simulink model "localization_and_state_estimation"  (R2023a)
settings: Solver=ode1  StartTime=0.0  StopTime=inf  FixedStep=1/60  RelTol=1e-3  EnableMultiTasking=on
model workspace (MAT data in the model file):
  downCamStepSize = Simulink.Parameter
  downCamStepSize.Value = Simulink.data.Expression
  downCamStepSize.Value.ExpressionString = "qc_get_step_size*ceil(1/60/qc_get_step_size)"
  downCamStepSize.DataType = 'auto'
  downCamStepSize.Complexity = 'real'
  downCamStepSize.Dimensions = -1
  lidarStepSize = Simulink.Parameter
  lidarStepSize.Value = Simulink.data.Expression
  lidarStepSize.Value.ExpressionString = "qc_get_step_size*ceil(1/5/qc_get_step_size)"
  lidarStepSize.DataType = 'auto'
  lidarStepSize.Complexity = 'real'
  lidarStepSize.Dimensions = -1
  mainStepSize = Simulink.Parameter
  mainStepSize.Value = Simulink.data.Expression
  mainStepSize.Value.ExpressionString = "qc_get_step_size"
  mainStepSize.DataType = 'auto'
  mainStepSize.Complexity = 'real'
  mainStepSize.Dimensions = -1
  mode = Simulink.Parameter
  mode.Value = 1
  mode.Description = '0 - education speeds via wheel speed commands
    | 1 - education speeds via body speed commands
    | 2 - research speeds via wheel speed commands
    | 3 - research speeds via body speed commands'
  mode.DataType = 'auto'
  mode.Complexity = 'real'
  mode.Dimensions = [1 1]
  realSenseStepSize = Simulink.Parameter
  realSenseStepSize.Value = Simulink.data.Expression
  realSenseStepSize.Value.ExpressionString = "qc_get_step_size*ceil(1/30/qc_get_step_size)"
  realSenseStepSize.DataType = 'auto'
  realSenseStepSize.Complexity = 'real'
  realSenseStepSize.Dimensions = -1
undefined symbols (not defined in the file): gcbh, JPEG, Point, video_display_show
libraries: quarc_library x33, simulink x2
(part 1 of 2)
settings Model: SimulationMode=external  ExtModeTrigDuration=10000  Creator=mbohra  LastModifiedBy=mbohra
settings SolverCC: AlgebraicLoopSolver=TrustRegion  PositivePriorityOrder=on
settings DataIOCC: ReturnWorkspaceOutputs=off
settings DebuggingCC: ParameterPrecisionLossMsg=none  UnconnectedInputMsg=warning  UnconnectedOutputMsg=warning  UnconnectedLineMsg=warning  ArithmeticOperatorsInVariantConditions=warning
settings HardwareCC: ProdBitPerLong=64  ProdLargestAtomicInteger=LongLong  ProdLargestAtomicFloat=Double  ProdLongLongMode=on  ProdHWDeviceType=ARM Compatible->ARM 64-bit (LP64)
settings ModelReferenceCC: EnableRefExpFcnMdlSchedulingChecks=on
settings SFSimCC: SimUseLocalCustomCode=off  CustomCodeUndefinedFunction=UseInterfaceOnly
settings RTWCC: Description=QUARC Linux QBot Platform Target Using Toolchain  SystemTargetFile=quarc_linux_qbot_platform.tlc  TemplateMakefile=quarc_default_tmf  RTWUseLocalCustomCode=off  Toolchain=QUARC linux_qbot_platform | gmake (64-bit Windows)  BuildConfiguration=Faster Runs
settings CodeAppCC: StateflowObjectComments=on
settings STFCustomTargetCC: SystemTargetFile=quarc_linux_qbot_platform.tlc
settings GRTTargetCC: ParMdlRefBuildCompliant=off  CompOptLevelCompliant=off  CombineOutputUpdateFcns=off  MatFileLogging=off  CPPClassGenCompliant=off  GRTInterface=on  ExtMode=on  ExtModeMexFile=quarc_comm  ExtModeMexArgs='-w -d /tmp -uri %u','tcpip://192.168.3.14:17001'
settings ConfigComp: CovMetricSettings=dswe

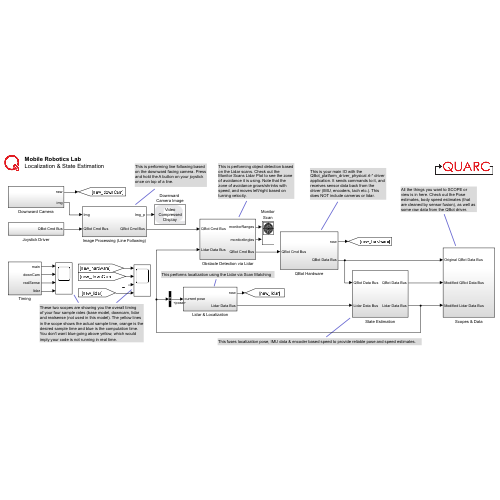
[thumbnail: Simulink's stored preview of the top-level diagram]
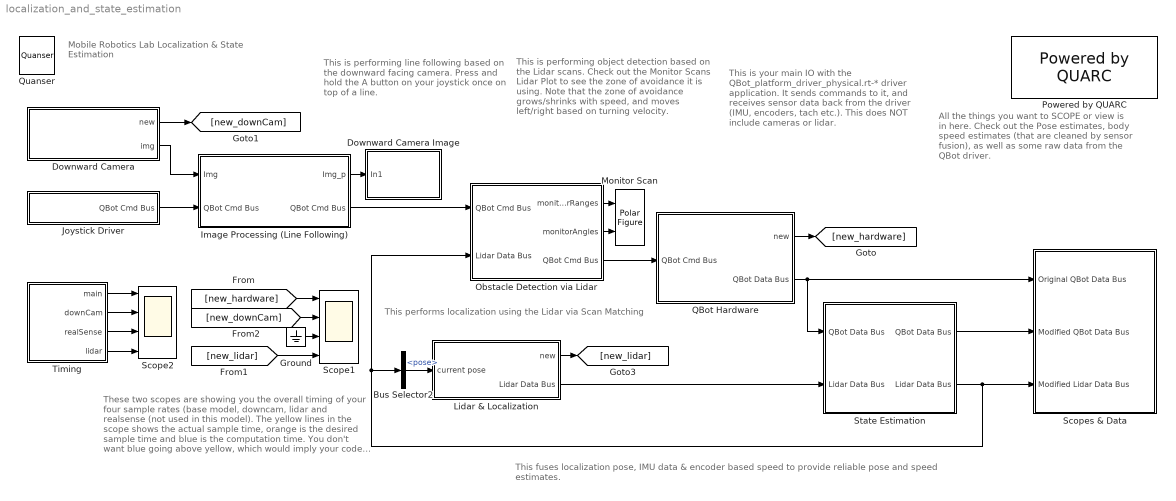
== system localization_and_state_estimation ==
  note: These two scopes are showing you the overall timing
      | of your four sample rates (base model, downcam, lidar
      | and realsense (not used in this model). The yellow lines
      | in the scope shows the actual sample time, orange is the
      | desired sample time and blue is the computation time.
      | You don't want blue going above yellow, which would
      | imply your code is not running in real time.
  note: This is performing line following based on the downward facing camera. Press and hold the A button on your joystick once on top of a line.
  note: Mobile Robotics Lab
      | Localization & State Estimation
  note: This is performing object detection based on the Lidar scans. Check out the Monitor Scans Lidar Plot to see the zone of avoidance it is using. Note that the zone of avoidance grows/shrinks with speed, and moves left/right based on turning velocity.
  note: This is your main IO with the QBot_platform_driver_physical.rt-* driver application. It sends commands to it, and receives sensor data back from the driver (IMU, encoders, tach etc.). This does NOT include cameras or lidar.
  note: All the things you want to SCOPE or view is in here. Check out the Pose estimates, body speed estimates (that are cleaned by sensor fusion), as well as some raw data from the QBot driver.
  note: This performs localization using the Lidar via Scan Matching
  note: This fuses localization pose, IMU data & encoder based speed to provide reliable pose and speed estimates.
  Bus Selector2 : BusSelector  OutputSignals=pose
  Downward Camera Image : Subsystem  LoadFcn=set_param(gcbh, 'UserData', gcb);  StartFcn=video_display_show([gcb, '/Video Display'], 'add', gcb);  mask(Video Compressed Display){algorithm=JPEG, quality=50, sample_time=-1, use_hardware=on}
      mask prompts: algorithm "Compression algorithm:"; quality "Compression quality (0-100):"; sample_time "Sample time (seconds):"; use_hardware "Use hardware acceleration for video display"
      mask help: Displays a video stream on the host, using compression to minimize bandwidth.
      mask init:
      | qc_set_display('Video\nCompressed\nDisplay');
      settings: UndoDeleteFcn=set_param(gcbh, 'UserData', gcb);  OpenFcn=video_display_show([gcb, '/Video Display'], 'show', gcb);  PreDeleteFcn=video_display_show([gcb, '/Video Display'], 'delete');
      settings: CopyFcn=|
      | set_param(gcbh, 'UserData', gcb);
      | set_param(gcbh, 'LinkStatus', 'none');
      settings: NameChangeFcn=|
      | video_display_show([get_param(gcbh, 'UserData'), '/Video Display'], 'rename', [gcb, '/Video Display']);
      | video_display_show([gcb, '/Video Display'], 'add', gcb);
      | set_param(gcbh, 'UserData', gcb);
      mask Help: web(qc_get_block_help_path(gcb));
      mask TypeOptions algorithm: Image Compress/algorithm
      mask TypeOptions quality: Image Compress/quality
      mask TypeOptions sample_time: Video Display/sample_time
      mask TypeOptions use_hardware: Video Display/use_hardware
      mask Display:
      | patch([0.98591 0.98591 0.62618 0.59072 0.56147   0.536   0.536  0.5441 0.56912 0.59207 0.60881 0.62276 0.63527 0.64364  0.6485  0.6485 0.64706 0.64499 0.63662 0.62411 0.61232 0.59837 0.58307 0.56147   0.536   0.536  0.5441  0.5747 0.60953 0.63662 0.67001  0.7034 0.72851 0.75425 0.77927 0.80294 0.82454 0.84119 0.85865 0.87395 0.88574 0.89339  0.8969 0.89969 0.89969 0.89267  0.8816 0.87044 0.85649  0.8384 0.81824 0.80294 0.78764 0.77513 0.76676 0.75776 0.76397 0.77513 0.79178 0.80987 0.82796 0.84326 0.86207 0.98528],[0.18689 0.05522 0.05522 0.05171 0.05171    0.05 0.18338 0.18338 0.19148 0.20435 0.22298 0.24863 0.28589 0.33125 0.38138 0.55139 0.59801 0.63761 0.68189 0.72149 0.74939 0.76694 0.77855 0.79367 0.79952 0.92768 0.92768 0.92768 0.92417 0.92066 0.91364  0.9032 0.89384 0.88106 0.86594 0.85073 0.82634 0.80537 0.77855 0.74363 0.70403 0.65858 0.61079 0.59099 0.41513 0.37202 0.31847 0.29048 0.25556 0.23342  0.2102 0.19382 0.18221 0.17285 0.16943 0.16124  0.1589 0.16241 0.16709 0.17168  0.1787 0.18221 0.18689 0.18689],[0.9,0.90,0.91])
      | patch([0.536 0.52601 0.46823 0.44528 0.41603 0.39101 0.35555 0.33116 0.31451 0.29291  0.2804 0.26717 0.25322 0.23999 0.22406 0.20732 0.19337 0.17528 0.15935 0.14396 0.13217 0.11759 0.10922 0.10085 0.09671 0.09392 0.09041 0.08906 0.08906 0.09464  0.0995 0.10778 0.11894 0.13145 0.14675 0.16349 0.17672 0.19409 0.20732 0.22406 0.23999 0.26159 0.27833 0.29849 0.31793 0.33602 0.35411 0.37085 0.39245 0.41603   0.536   0.536 0.53159 0.46409   0.446 0.42026 0.39587 0.37571 0.36113 0.34925 0.34088 0.33809 0.33809 0.34088 0.34583 0.35627 0.36392 0.38129 0.39587 0.41117 0.42719 0.44672  0.4676 0.48353 0.48353 0.52394   0.536],[0.05 0.04829 0.04712 0.04712 0.04829 0.05063 0.05405 0.05873 0.06107 0.06692 0.07043 0.07619 0.08087 0.08672 0.09482 0.10652 0.11696 0.13325  0.1508 0.17168 0.19499 0.22415 0.25439 0.28472 0.31379 0.35456 0.38489 0.41513 0.58055 0.63878 0.68774 0.72149 0.75641 0.78089 0.80537 0.82859 0.84029 0.85658 0.86594 0.87404  0.8834 0.89267 0.90086 0.90788 0.91247 0.91832 0.92066   0.923 0.92651 0.92768 0.92768 0.79952 0.79952 0.79952 0.79718 0.78899 0.77153 0.75056 0.72149 0.68072 0.62249  0.5549 0.41396 0.37085 0.33242 0.28121 0.25205 0.22181 0.20552 0.19499 0.18572 0.18221 0.17753 0.17636 0.17753  0.1787  0.1787],[0.9,0.90,0.91])
      | disp('Video\nCompressed\nDisplay');
  Downward Camera : Subsystem
  Ground : Ground
  Image Processing (Line Following) : Subsystem
  Joystick Driver : Subsystem
  Lidar & Localization : Subsystem
  Monitor Scan : quarc_library/Sinks/Figures/Polar Figure  figure_mode=Use figure window  figure_tag=figure1  axes_tag=axes1  plot_mode=Frame-based  minimum_rho=0  maximum_rho=4  minimum_theta=0  maximum_theta=360  zero_location=top  direction=counterclockwise  buffer_size=2  update_rate=1  sample_time=-1  initial_position="1290    55   483   448"  initial_visibility=off  line1_style=None  line1_width=0.5  line1_color=[0 0 0]  marker1=Point (.)  marker1_size=6  marker1_edge_color=[0 0 0]  marker1_face_color=[0 0 0]  line2_style=Solid line (-)  line2_width=0.5  line2_color=[0.85098 0.32549 0.0980392]  marker2=None  marker2_size=6  marker2_edge_color=[0.85098 0.32549 0.0980392]  marker2_face_color=[0.85098 0.32549 0.0980392]  line3_style=Solid line (-)  line3_width=0.5  line3_color=[0.929412 0.694118 0.12549]  marker3=None  marker3_size=6  marker3_edge_color=[0.929412 0.694118 0.12549]  marker3_face_color=[0.929412 0.694118 0.12549]  line4_style=Solid line (-)  line4_width=0.5  line4_color=[0.494118 0.184314 0.556863]  marker4=None  marker4_size=6  marker4_edge_color=[0.494118 0.184314 0.556863]  marker4_face_color=[0.494118 0.184314 0.556863]  line5_style=Solid line (-)  line5_width=0.5  line5_color=[0.466667 0.67451 0.188235]  marker5=None  marker5_size=6  marker5_edge_color=[0.466667 0.67451 0.188235]  marker5_face_color=[0.466667 0.67451 0.188235]
      settings: SourceProductName=QUARC Targets
  Obstacle Detection via Lidar : Subsystem
  Powered by QUARC : quarc_library/Logos/Powered by QUARC
  QBot Hardware : Subsystem
  Quanser : quarc_library/Logos/Quanser
  Scope1 : Scope  NumInputPorts=4
  Scope2 : Scope  NumInputPorts=4
  Scopes & Data : Subsystem
  State Estimation : Subsystem
  Timing : Subsystem
  wires:
  QBot Hardware/2(QBot Data Bus) -> Scopes & Data/1(Original QBot Data Bus), State Estimation/1("QBot Data Bus ")
  QBot Hardware/1(new) -> [new_hardware]
  Lidar & Localization/1(new) -> [new_lidar]
  [new_downCam] -> Scope1/2
  Timing/3(realSense) -> Scope2/3
  Timing/4(lidar) -> Scope2/4
  [new_lidar] -> Scope1/4
  Timing/2(downCam) -> Scope2/2
  [new_hardware] -> Scope1/1
  Timing/1(main) -> Scope2/1
  Obstacle Detection via Lidar/1(monitorRanges) -> Monitor Scan/1
  Obstacle Detection via Lidar/2(monitorAngles) -> Monitor Scan/2
  Obstacle Detection via Lidar/3(QBot Cmd Bus) -> QBot Hardware/1(QBot Cmd Bus)
  Downward Camera/2(img) -> Image Processing (Line Following)/1(Img)
  Joystick Driver/1(QBot Cmd Bus) -> Image Processing (Line Following)/2(QBot Cmd Bus)
  Image Processing (Line Following)/1(Img_p) -> Downward Camera Image/1(In1)
  Image Processing (Line Following)/2(" QBot Cmd Bus") -> Obstacle Detection via Lidar/1("QBot Cmd Bus ")
  Downward Camera/1(new) -> [new_downCam]
  Ground/1 -> Scope1/3
  Lidar & Localization/2(Lidar Data Bus) -> State Estimation/2("Lidar Data Bus ")
  State Estimation/2(Lidar Data Bus) -> Bus Selector2/1, Obstacle Detection via Lidar/2(Lidar Data Bus), Scopes & Data/3(Modified Lidar Data Bus)
  Bus Selector2/1 -> Lidar & Localization/1(current pose)  "<pose>"
  State Estimation/1(QBot Data Bus) -> Scopes & Data/2(Modified QBot Data Bus)

== system localization_and_state_estimation/Downward Camera Image ==
  In1 : Inport
  Channel : quarc_library/Signal Routing/Channel  channel=0  buffer_size=1
  Image Compress : quarc_library/Image Processing/Generic/Image Compress  algorithm=JPEG  source=Internal dialog parameter  quality=quality  output_dim=-1
  Video Display : quarc_library/Multimedia/Video Display  Tag="localization_and_state_estimation/Downward  Camera Image/Video Display"  sample_time=sample_time  use_hardware=on
  wires:
  Channel/1 -> Video Display/1
  In1/1 -> Image Compress/1
  Image Compress/1 -> Channel/1

== system localization_and_state_estimation/Downward Camera ==
  Rate Transition : RateTransition
  Video Capture : quarc_library/Multimedia/Video Capture  source=device  device=0  filename=sample_movie.mov  value=[0 0; 0 0]  resolution=640 x 400  width=640  height=400  output_format=MATLAB greyscale (HxW)  data_type=uint8  sample_time=downCamStepSize  brightness_override=off  brightness=50.0  contrast_override=off  contrast=50.0  hue_override=off  hue=50.0  saturation_override=off  saturation=50.0  sharpness_override=off  sharpness=50.0  gamma_override=off  gamma=50.0  coloreffect_override=off  coloreffect=None  whitebalance_override=off  whitebalance=50.0  backlightcompensation_override=off  backlightcompensation=0.0  gain_override=on  gain=17.0  pan_override=off  pan=50.0  tilt_override=off  tilt=50.0  roll_override=off  roll=50.0  zoom_override=off  zoom=0.0  exposure_override=on  exposure=39.0  iris_override=off  iris=50.0  mirror_override=off  mirror=None  focus_override=off  focus=0.0
      settings: SourceProductName=QUARC Targets
  new : Outport
  img : Outport  Port=2
  wires:
  Video Capture/2 -> Rate Transition/1
  Video Capture/1 -> img/1
  Rate Transition/1 -> new/1

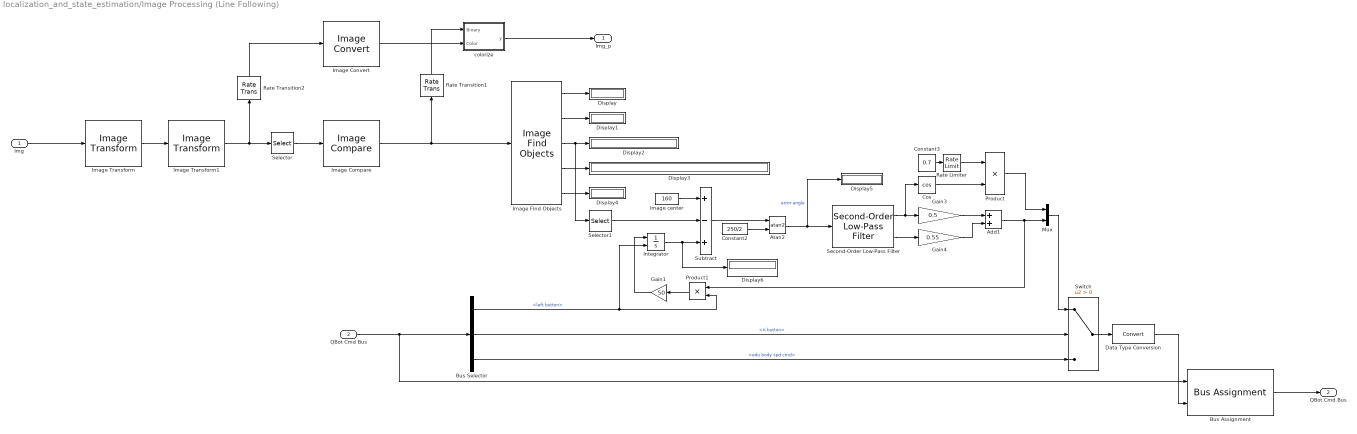
== system localization_and_state_estimation/Image Processing (Line Following) ==
  Img : Inport
  QBot Cmd Bus : Inport  Port=2
  Add1 : Sum
  Atan2 : Trigonometry  Operator=atan2
  Bus Assignment : BusAssignment  AssignedSignals=edu body spd cmd
  Bus Selector : BusSelector  OutputSignals=left button,A button,edu body spd cmd
  Constant2 : Constant  Value=250/2
  Constant3 : Constant  Value=0.7
  Cos : Trigonometry  Operator=cos
  Data Type Conversion : DataTypeConversion  SaturateOnIntegerOverflow=off  RndMeth=Floor
  Display{,1..6} (7 alike) : Display
      Display settings: Format=bank
      Display1 settings: Format=bank
      Display2 settings: Format=bank
      Display3 settings: Format=bank
      Display4 settings: Format=bank
  Gain1 : Gain  Gain=50
  Gain3 : Gain  Gain=0.5
  Gain4 : Gain  Gain=0.55
  Image Compare : quarc_library/Image Processing/Generic/Image Compare  output_type=Combined (one HxW output)  source=Internal dialog parameters  r_comparison=min <= pixel and pixel <= max  r_minimum=225  r_maximum=255  g_comparison=min <= pixel and pixel <= max  g_minimum=225  g_maximum=255  b_comparison=min <= pixel and pixel <= max  b_minimum=225  b_maximum=255
      settings: SourceProductName=QUARC Targets
  Image Convert : quarc_library/Image Processing/Generic/Image Convert  input_format=MATLAB greyscale (HxW)  padding=0  output_format=MATLAB RGB (HxWx3)  data_type=uint8
      settings: AttributesFormatString=(%<input_format>)  SourceProductName=QUARC Targets
  Image Find Objects : quarc_library/Image Processing/Generic/Image Find Objects  num_objects=1  connectivity=8 directions (N, NE, E, SE, S, SW, W, NW)  sort_order=Sort by number of pixels  min_pixels=500  max_pixels=intmax('uint32')  largest=on  exclude_at_edges=off  variable_size=off  use_complex=off
      settings: SourceProductName=QUARC Targets
  Image Transform : quarc_library/Image Processing/Generic/Image Transform  algorithm=Lens undistort  color_theme=KRYGCBMW  min_pixel=0  max_pixel=4000  focal_length=[302.1629, 301.7493]  principal_point=[185.6271, 306.7551]  radial_coeffs=[-0.3138 0.0780]  tangential_coeffs=[]  extrapolated_pixel=0  interpolation=nearest  row_coords=0  column_coords=0  output_height=480  output_width=640  angle=0  origin=[240 320]  output_origin=[240 320]  output_data_type=uint8
      settings: AttributesFormatString=(%<algorithm>)  SourceProductName=QUARC Targets
  Image Transform1 : quarc_library/Image Processing/Generic/Image Transform  algorithm=Resize  color_theme=KRYGCBMW  min_pixel=0  max_pixel=4000  focal_length=308  principal_point=[262 334]  radial_coeffs=[-0.3129 0.0907]  tangential_coeffs=[]  extrapolated_pixel=0  interpolation=nearest  row_coords=0  column_coords=0  output_height=200  output_width=320  angle=0  origin=[240 320]  output_origin=[240 320]  output_data_type=uint8
      settings: AttributesFormatString=(%<algorithm>)  SourceProductName=QUARC Targets
  Image center : Constant  Value=160
  Integrator : Integrator  ExternalReset=falling  LimitOutput=on  UpperSaturationLimit=160  LowerSaturationLimit=-160
  Mux : Mux  Inputs=2
  Product : Product
  Product1 : Product
  Rate Limiter : RateLimiter  SampleTimeMode=inherited
  Rate Transition1 : RateTransition  OutPortSampleTime=downCamStepSize*2
  Rate Transition2 : RateTransition  OutPortSampleTime=downCamStepSize*2
  Second-Order Low-Pass Filter : quarc_library/Continuous/Second-Order Low-Pass Filter  params_source=Internal (dialog parameters)  input_width=2*pi*5  input_zeta=1  input_init=0
  Selector : Selector  NumberOfDimensions=2  InputPortWidth=3  IndexOptions=Index vector (dialog),Select all  Indices=[51:100],[101:540]  OutputSizes=1,1
  Selector1 : Selector  InputPortWidth=2  IndexOptions=Index vector (dialog)  Indices=2  OutputSizes=1
  Subtract : Sum  Inputs=+-+
  Switch : Switch  Criteria=u2 > Threshold  SaturateOnIntegerOverflow=off  InputSameDT=off
  colorize : MATLAB Function  TreatAsAtomicUnit=on
  Img_p : Outport
  " QBot Cmd Bus" : Outport  Port=2
  wires:
  Selector1/1 -> Subtract/2
  Image center/1 -> Subtract/1
  Image Find Objects/5 -> Display4/1
  Image Find Objects/3 -> Display2/1, Selector1/1
  Image Find Objects/4 -> Display3/1
  Image Find Objects/2 -> Display1/1
  Image Find Objects/1 -> Display/1
  Image Compare/1 -> Image Find Objects/1, Rate Transition1/1
  Image Transform1/1 -> Rate Transition2/1, Selector/1
  Selector/1 -> Image Compare/1
  Rate Transition1/1 -> colorize/1(Binary)
  Atan2/1 -> Display5/1, Second-Order Low-Pass Filter/1  "error angle"
  Subtract/1 -> Atan2/1
  Constant2/1 -> Atan2/2
  Cos/1 -> Product/2
  Constant3/1 -> Rate Limiter/1
  Product/1 -> Mux/1
  Mux/1 -> Switch/1
  Add1/1 -> Product1/1, Mux/2
  Integrator/1 -> Display6/1, Subtract/3
  Gain1/1 -> Integrator/1
  Bus Selector/1 -> Integrator/2, Product1/2  "<left button>"
  Gain4/1 -> Add1/2
  Gain3/1 -> Add1/1
  Second-Order Low-Pass Filter/2 -> Gain4/1
  Second-Order Low-Pass Filter/1 -> Cos/1, Gain3/1
  Product1/1 -> Gain1/1
  Rate Transition2/1 -> Image Convert/1
  colorize/1(y) -> Img_p/1
  Image Convert/1 -> colorize/2(Color)
  Image Transform/1 -> Image Transform1/1
  Img/1 -> Image Transform/1
  QBot Cmd Bus/1 -> Bus Assignment/1, Bus Selector/1
  Bus Selector/3 -> Switch/3  "<edu body spd cmd>"
  Bus Selector/2 -> Switch/2  "<A button>"
  Switch/1 -> Data Type Conversion/1
  Bus Assignment/1 -> " QBot Cmd Bus"/1
  Data Type Conversion/1 -> Bus Assignment/2
  Rate Limiter/1 -> Product/1

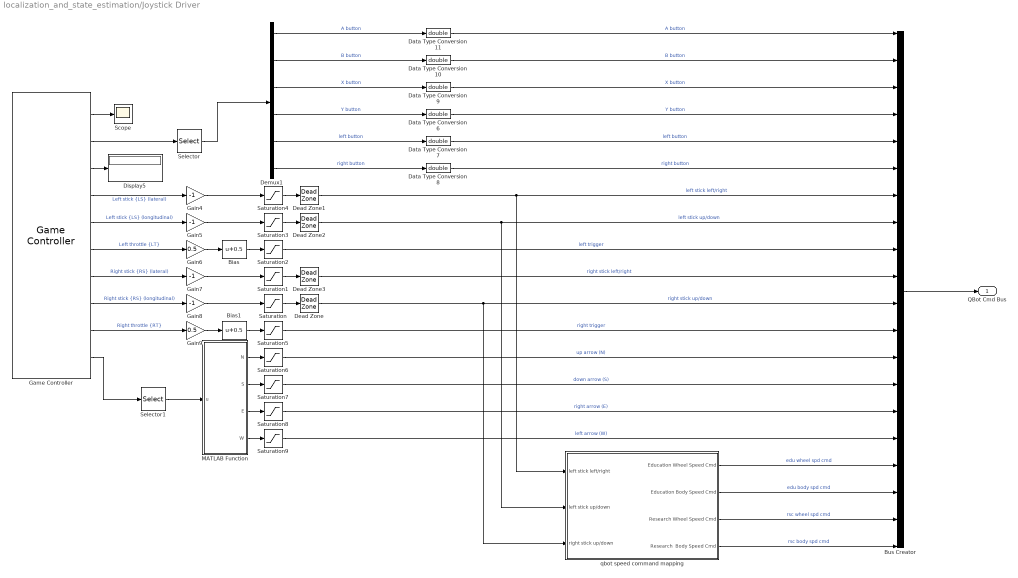
== system localization_and_state_estimation/Joystick Driver ==
  Bias : Bias  Bias=0.5  SaturateOnIntegerOverflow=off
  Bias1 : Bias  Bias=0.5  SaturateOnIntegerOverflow=off
  Bus Creator : BusCreator  Inputs=20
  Data Type Conversion{6..11} (6 alike) : DataTypeConversion  OutDataTypeStr=double  SaturateOnIntegerOverflow=off  RndMeth=Floor
  Dead Zone{,1..3} (4 alike) : DeadZone  LowerValue=-0.05  UpperValue=0.05
  Demux1 : Demux  Outputs=6
  Display5 : Display
  Gain{4..5,7..8} (4 alike) : Gain  Gain=-1
  Gain6 : Gain  Gain=0.5
  Gain9 : Gain  Gain=0.5
  Game Controller : quarc_library/Devices/Peripherals/Target/Game Controller  controller=1  buffer_size=12  deadzone=[]  saturation=[]  sample_time=qc_get_step_size  auto_center=off  enabled=on
      settings: SourceProductName=QUARC Targets
  MATLAB Function : MATLAB Function  TreatAsAtomicUnit=on
  Saturation{,1,3..4} (4 alike) : Saturate  UpperLimit=1  LowerLimit=-1
  Saturation{2,5..9} (6 alike) : Saturate  UpperLimit=1  LowerLimit=0
  Scope : Scope
  Selector : Selector  InputPortWidth=32  IndexOptions=Index vector (dialog)  Indices=[1:6]  OutputSizes=1
  Selector1 : Selector  InputPortWidth=4  IndexOptions=Index vector (dialog)  Indices=1  OutputSizes=1
  qbot speed command mapping : Subsystem
  QBot Cmd Bus : Outport
  wires:
  Game Controller/1 -> Scope/1
  Game Controller/2 -> Selector/1
  Game Controller/3 -> Display5/1
  Game Controller/4 -> Gain4/1  "Left stick {LS} (lateral)"
  Game Controller/5 -> Gain5/1  "Left stick {LS} (longitudinal)"
  Game Controller/6 -> Gain6/1  "Left throttle {LT}"
  Game Controller/7 -> Gain7/1  "Right stick {RS} (lateral)"
  Game Controller/8 -> Gain8/1  "Right stick {RS} (longitudinal)"
  Game Controller/9 -> Gain9/1  "Right throttle {RT}"
  Game Controller/10 -> Selector1/1
  Selector/1 -> Demux1/1
  Selector1/1 -> MATLAB Function/1(u)
  Gain6/1 -> Bias/1
  Gain9/1 -> Bias1/1
  Gain8/1 -> Saturation/1
  Gain7/1 -> Saturation1/1
  Gain5/1 -> Saturation3/1
  Gain4/1 -> Saturation4/1
  Bias/1 -> Saturation2/1
  Bias1/1 -> Saturation5/1
  Saturation4/1 -> Dead Zone1/1
  Saturation3/1 -> Dead Zone2/1
  Saturation1/1 -> Dead Zone3/1
  Saturation/1 -> Dead Zone/1
  MATLAB Function/1(N) -> Saturation6/1
  MATLAB Function/2(S) -> Saturation7/1
  MATLAB Function/3(E) -> Saturation8/1
  MATLAB Function/4(W) -> Saturation9/1
  Demux1/5 -> Data Type Conversion7/1  "left button"
  Demux1/6 -> Data Type Conversion8/1  "right button"
  Dead Zone/1 -> qbot speed command mapping/3(right stick up/down), Bus Creator/11  "right stick up/down"
  Dead Zone1/1 -> qbot speed command mapping/1(left stick left/right), Bus Creator/7  "left stick left/right"
  Demux1/4 -> Data Type Conversion6/1  "Y button"
  Demux1/3 -> Data Type Conversion9/1  "X button"
  Demux1/2 -> Data Type Conversion10/1  "B button"
  Demux1/1 -> Data Type Conversion11/1  "A button"
  Dead Zone2/1 -> qbot speed command mapping/2(left stick up/down), Bus Creator/8  "left stick up/down"
  Saturation6/1 -> Bus Creator/13  "up arrow (N)"
  Saturation7/1 -> Bus Creator/14  "down arrow (S)"
  Saturation8/1 -> Bus Creator/15  "right arrow (E)"
  Saturation9/1 -> Bus Creator/16  "left arrow (W)"
  qbot speed command mapping/1(Education Wheel Speed Cmd) -> Bus Creator/17  "edu wheel spd cmd"
  qbot speed command mapping/2(Education Body Speed Cmd) -> Bus Creator/18  "edu body spd cmd"
  qbot speed command mapping/3(Research Wheel Speed Cmd) -> Bus Creator/19  "rsc wheel spd cmd"
  qbot speed command mapping/4(Research  Body Speed Cmd) -> Bus Creator/20  "rsc body spd cmd"
  Saturation2/1 -> Bus Creator/9  "left trigger"
  Dead Zone3/1 -> Bus Creator/10  "right stick left/right"
  Saturation5/1 -> Bus Creator/12  "right trigger"
  Bus Creator/1 -> QBot Cmd Bus/1
  Data Type Conversion6/1 -> Bus Creator/4  "Y button"
  Data Type Conversion8/1 -> Bus Creator/6  "right button"
  Data Type Conversion7/1 -> Bus Creator/5  "left button"
  Data Type Conversion9/1 -> Bus Creator/3  "X button"
  Data Type Conversion10/1 -> Bus Creator/2  "B button"
  Data Type Conversion11/1 -> Bus Creator/1  "A button"

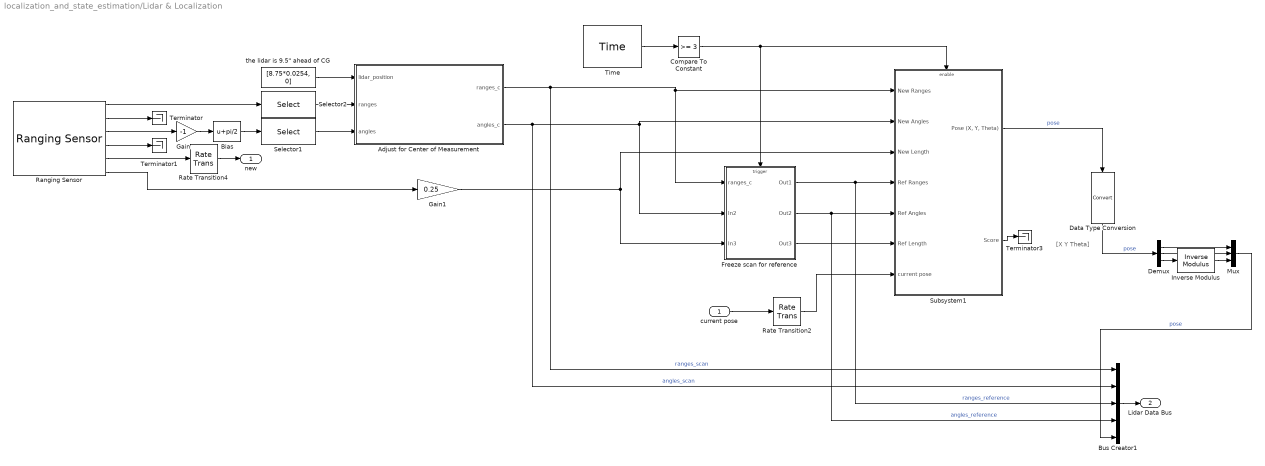
== system localization_and_state_estimation/Lidar & Localization ==
  note: [X Y Theta]
  current pose : Inport
  Adjust for Center of Measurement : MATLAB Function  TreatAsAtomicUnit=on  SystemSampleTime=lidarStepSize
  Bias : Bias  Bias=pi/2  SaturateOnIntegerOverflow=off
  Bus Creator1 : BusCreator  Inputs=5
  Compare To Constant : simulink/Logic and Bit Operations/Compare To Constant  relop=>=  const=3  OutDataTypeStr=boolean
  Data Type Conversion : DataTypeConversion  SaturateOnIntegerOverflow=off  RndMeth=Floor
  Demux : Demux  Outputs=3
  Freeze scan for reference : Subsystem  TreatAsAtomicUnit=on
  Gain : Gain  Gain=-1
  Gain1 : Gain  Gain=0.25  OutDataTypeStr=int32
  Inverse Modulus : quarc_library/Discontinuities/Inverse Modulus  modulus=2*pi  output_derivative=off  output_revolutions=off  max_x=Inf  min_x=-Inf
  Mux : Mux  Inputs=3
  Ranging Sensor : quarc_library/Devices/Third-Party/Sensors/Ranging Sensor  sensor_type=Leishen M10P LIDAR  uri=serial://localhost:0?device='/dev/lidar',baud='512000',word='8',parity='none',stop='1',flow='none'  ranging_distance=Short  timing_budget=0.033  measurement_period=0.0005  output_mode=Fixed-size output  samples_per_revolution=1680  max_distance=0.050  max_angle=5  sample_time=lidarStepSize  show_versions=off  active=on
      settings: SourceProductName=QUARC Targets
  Rate Transition2 : RateTransition
  Rate Transition4 : RateTransition
  Selector1 : Selector  InputPortWidth=1680  IndexOptions=Index vector (dialog)  Indices=[1:4:1677]  OutputSizes=1
  Selector2 : Selector  InputPortWidth=1680  IndexOptions=Index vector (dialog)  Indices=[1:4:1677]  OutputSizes=1
  Subsystem1 : Subsystem
  Terminator : Terminator
  Terminator1 : Terminator
  Terminator3 : Terminator
  Time : quarc_library/Sources/Time/Time  time_source=Wall clock  sample_time=lidarStepSize
  "the lidar is 9.5\" ahead of CG" : Constant  Value=[8.75*0.0254, 0]  SampleTime=lidarStepSize
  new : Outport
  Lidar Data Bus : Outport  Port=2
  wires:
  Ranging Sensor/5 -> Rate Transition4/1
  Rate Transition4/1 -> new/1
  Selector1/1 -> Adjust for Center of Measurement/3(angles)
  Selector2/1 -> Adjust for Center of Measurement/2(ranges)
  "the lidar is 9.5\" ahead of CG"/1 -> Adjust for Center of Measurement/1(lidar_position)
  Bias/1 -> Selector1/1
  Ranging Sensor/2 -> Terminator/1
  Ranging Sensor/4 -> Terminator1/1
  Gain/1 -> Bias/1
  Ranging Sensor/3 -> Gain/1
  Ranging Sensor/1 -> Selector2/1
  Ranging Sensor/6 -> Gain1/1
  Compare To Constant/1 -> Subsystem1/Enable, Freeze scan for reference/Trigger
  Subsystem1/1("Pose (X, Y, Theta)") -> Data Type Conversion/1  "pose"
  Freeze scan for reference/3(Out3) -> Subsystem1/6(Ref Length)
  Adjust for Center of Measurement/2(angles_c) -> Freeze scan for reference/2(In2), Subsystem1/2(New Angles), Bus Creator1/2  "angles_scan"
  Freeze scan for reference/2(Out2) -> Bus Creator1/4, Subsystem1/5(Ref Angles)  "angles_reference"
  Gain1/1 -> Subsystem1/3(New Length), Freeze scan for reference/3(In3)
  Adjust for Center of Measurement/1(ranges_c) -> Subsystem1/1(New Ranges), Freeze scan for reference/1(ranges_c), Bus Creator1/1  "ranges_scan"
  Time/1 -> Compare To Constant/1
  Bus Creator1/1 -> Lidar Data Bus/1
  Freeze scan for reference/1(Out1) -> Bus Creator1/3, Subsystem1/4(Ref Ranges)  "ranges_reference"
  Subsystem1/2(Score) -> Terminator3/1
  current pose/1 -> Rate Transition2/1
  Data Type Conversion/1 -> Demux/1  "pose"
  Rate Transition2/1 -> Subsystem1/7(current pose)
  Demux/2 -> Mux/2
  Demux/3 -> Inverse Modulus/1
  Demux/1 -> Mux/1
  Mux/1 -> Bus Creator1/5  "pose"
  Inverse Modulus/1 -> Mux/3

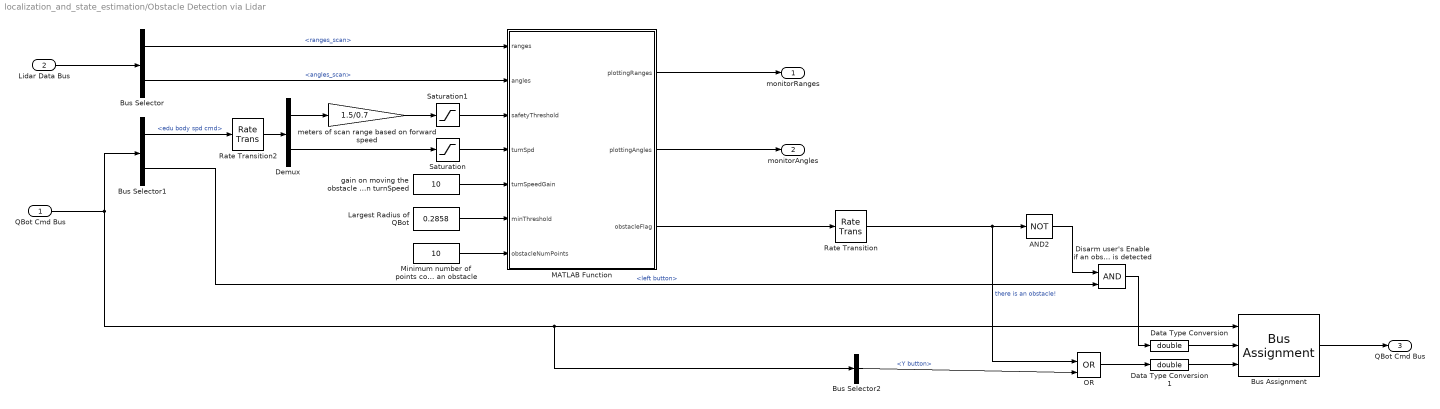
== system localization_and_state_estimation/Obstacle Detection via Lidar ==
  "QBot Cmd Bus " : Inport
  Lidar Data Bus : Inport  Port=2
  AND2 : Logic  Operator=NOT  IconShape=distinctive  AllPortsSameDT=off  OutDataTypeStr=boolean
  Bus Assignment : BusAssignment  AssignedSignals=left button,Y button
  Bus Selector : BusSelector  OutputSignals=ranges_scan,angles_scan
  Bus Selector1 : BusSelector  OutputSignals=edu body spd cmd,left button
  Bus Selector2 : BusSelector  OutputSignals=Y button
  Data Type Conversion : DataTypeConversion  OutDataTypeStr=double  SaturateOnIntegerOverflow=off  RndMeth=Floor
  Data Type Conversion1 : DataTypeConversion  OutDataTypeStr=double  SaturateOnIntegerOverflow=off  RndMeth=Floor
  Demux : Demux  Outputs=2
  Disarm user's Enable if an obstacle is detected : Logic  IconShape=distinctive  AllPortsSameDT=off  OutDataTypeStr=boolean
  Largest Radius of QBot : Constant  Value=0.2858
  MATLAB Function : MATLAB Function  TreatAsAtomicUnit=on
  Minimum number of points considered as an obstacle : Constant  Value=10
  OR : Logic  Operator=OR  IconShape=distinctive  AllPortsSameDT=off  OutDataTypeStr=boolean
  Rate Transition : RateTransition
  Rate Transition2 : RateTransition
  Saturation : Saturate  UpperLimit=3.564  LowerLimit=-3.564
  Saturation1 : Saturate  UpperLimit=2  LowerLimit=0.3
  "gain on moving the obstacle scan area left and right based on turnSpeed " : Constant  Value=10
  meters of scan range based on forward speed : Gain  Gain=1.5/0.7
  monitorRanges : Outport
  monitorAngles : Outport  Port=2
  QBot Cmd Bus : Outport  Port=3
  wires:
  Lidar Data Bus/1 -> Bus Selector/1
  Bus Selector/1 -> MATLAB Function/1(ranges)  "<ranges_scan>"
  Bus Selector/2 -> MATLAB Function/2(angles)  "<angles_scan>"
  Bus Selector1/1 -> Rate Transition2/1  "<edu body spd cmd>"
  Saturation1/1 -> MATLAB Function/3(safetyThreshold)
  MATLAB Function/3(obstacleFlag) -> Rate Transition/1
  Demux/2 -> Saturation/1
  Demux/1 -> meters of scan range based on forward speed/1
  Minimum number of points considered as an obstacle/1 -> MATLAB Function/7(obstacleNumPoints)
  meters of scan range based on forward speed/1 -> Saturation1/1
  MATLAB Function/1(plottingRanges) -> monitorRanges/1
  MATLAB Function/2(plottingAngles) -> monitorAngles/1
  "QBot Cmd Bus "/1 -> Bus Selector1/1, Bus Selector2/1, Bus Assignment/1
  Saturation/1 -> MATLAB Function/4(turnSpd)
  Rate Transition2/1 -> Demux/1
  AND2/1 -> Disarm user's Enable if an obstacle is detected/1
  Bus Selector1/2 -> Disarm user's Enable if an obstacle is detected/2  "<left button>"
  Bus Assignment/1 -> QBot Cmd Bus/1
  Disarm user's Enable if an obstacle is detected/1 -> Data Type Conversion/1
  Rate Transition/1 -> OR/1, AND2/1  "there is an obstacle!"
  Data Type Conversion/1 -> Bus Assignment/2
  Data Type Conversion1/1 -> Bus Assignment/3
  "gain on moving the obstacle scan area left and right based on turnSpeed "/1 -> MATLAB Function/5(turnSpeedGain)
  Largest Radius of QBot/1 -> MATLAB Function/6(minThreshold)
  Bus Selector2/1 -> OR/2  "<Y button>"
  OR/1 -> Data Type Conversion1/1

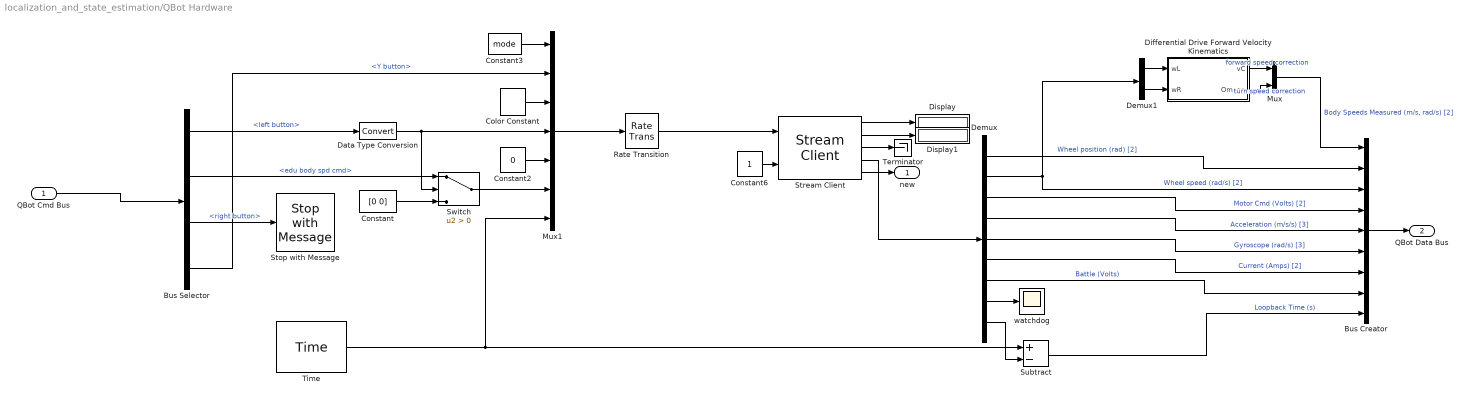
== system localization_and_state_estimation/QBot Hardware ==
  QBot Cmd Bus : Inport
  Bus Creator : BusCreator  Inputs=9
  Bus Selector : BusSelector  OutputSignals=left button,edu body spd cmd,right button,Y button
  Color Constant : quarc_library/Sources/Signals/Color Constant  color=[1 0 1]
      settings: SourceProductName=QUARC Targets
  Constant : Constant  Value=[0 0]
  Constant2 : Constant  Value=0
  Constant3 : Constant  Value=mode
  Constant6 : Constant
  Data Type Conversion : DataTypeConversion  SaturateOnIntegerOverflow=off  RndMeth=Floor
  Demux : Demux  Outputs=[2 2 2 3 3 2 1 1 1]
  Demux1 : Demux  Outputs=2
  Differential Drive Forward Velocity Kinematics : MATLAB Function  TreatAsAtomicUnit=on
  Display : Display
  Display1 : Display
  Mux : Mux  Inputs=2
  Mux1 : Mux  Inputs=7
  Rate Transition : RateTransition
  Stop with Message : quarc_library/Sinks/Error Handling/Stop with Message  message_type=Fixed error message  message_icon=Information  message=Operator: Emergency Stop
  Stream Client : quarc_library/Communications/Basic/Stream Client  uri_source=Specify via dialog (do not evaluate)  uri=tcpip://localhost:18888  send_buffer_size=1460  receive_buffer_size=1460  byte_order=little endian (Intel - LSB first)  optimization=Minimum latency  send_options=Send most recent data  receive_options=Receive most recent data  default_value=zeros(17,1)  sample_time=qc_get_step_size  active=off  implementation=Use blocking I/O in a separate thread  send_fifo_size=1000  receive_fifo_size=1000  send_priority=0  receive_priority=0  send_dimensions=off  receive_dimensions=off  max_dimensions=-1  data_type=Inherited via back propagation  type_expr=BusObject
      settings: AttributesFormatString="\"tcpip://localhost:18888\""
  Subtract : Sum  Inputs=+-
  Switch : Switch  Criteria=u2 > Threshold  SaturateOnIntegerOverflow=off  InputSameDT=off
  Terminator : Terminator
  Time : quarc_library/Sources/Time/Time  time_source=Wall clock  sample_time=qc_get_step_size
  watchdog : Scope
  new : Outport
  QBot Data Bus : Outport  Port=2
  wires:
  Constant3/1 -> Mux1/1
  Stream Client/3 -> Terminator/1
  Bus Selector/2 -> Switch/1  "<edu body spd cmd>"
  Stream Client/1 -> Display/1
  Constant6/1 -> Stream Client/2
  Stream Client/2 -> Display1/1
  Color Constant/1 -> Mux1/3
  Demux/3 -> Bus Creator/4  "Motor Cmd (Volts) [2]"
  Mux1/1 -> Rate Transition/1
  Stream Client/4 -> Demux/1
  Demux/1 -> Bus Creator/2  "Wheel position (rad) [2]"
  Stream Client/5 -> new/1
  Demux/7 -> Bus Creator/8  "Battle (Volts)"
  Demux/5 -> Bus Creator/6  "Gyroscope (rad/s) [3]"
  Demux/6 -> Bus Creator/7  "Current (Amps) [2]"
  Demux/9 -> Subtract/2
  Constant2/1 -> Mux1/5
  Demux/4 -> Bus Creator/5  "Acceleration (m/s/s) [3]"
  Time/1 -> Subtract/1, Mux1/7
  Bus Creator/1 -> QBot Data Bus/1
  Subtract/1 -> Bus Creator/9  "Loopback Time (s)"
  Demux/8 -> watchdog/1
  Switch/1 -> Mux1/6
  Constant/1 -> Switch/3
  QBot Cmd Bus/1 -> Bus Selector/1
  Bus Selector/3 -> Stop with Message/1  "<right button>"
  Bus Selector/1 -> Data Type Conversion/1  "<left button>"
  Data Type Conversion/1 -> Switch/2, Mux1/4
  Bus Selector/4 -> Mux1/2  "<Y button>"
  Demux/2 -> Demux1/1, Bus Creator/3  "Wheel speed (rad/s) [2]"
  Demux1/2 -> Differential Drive Forward Velocity Kinematics/2(wR)
  Demux1/1 -> Differential Drive Forward Velocity Kinematics/1(wL)
  Differential Drive Forward Velocity Kinematics/2(Omega) -> Mux/2  "turn speed correction"
  Differential Drive Forward Velocity Kinematics/1(vC) -> Mux/1  "forward speed correction"
  Mux/1 -> Bus Creator/1  "Body Speeds Measured (m/s, rad/s) [2]"
  Rate Transition/1 -> Stream Client/1

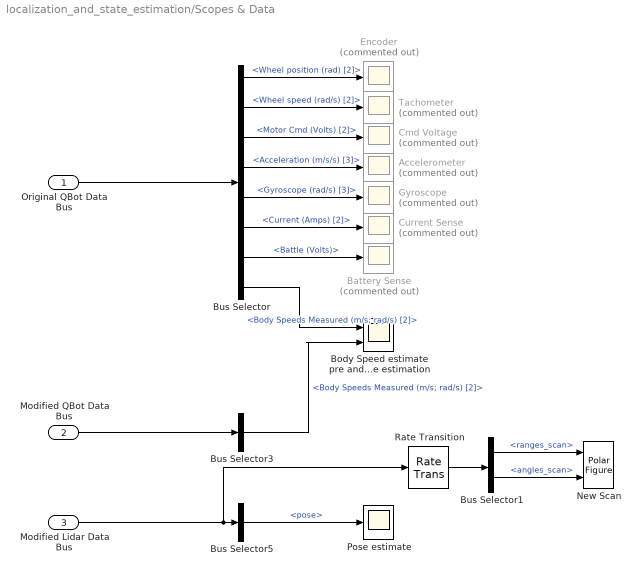
== system localization_and_state_estimation/Scopes & Data ==
  Original QBot Data Bus : Inport
  Modified QBot Data Bus : Inport  Port=2
  Modified Lidar Data Bus : Inport  Port=3
  Accelerometer : Scope  Commented=on
  Battery Sense : Scope  Commented=on
  Body Speed estimate pre and post state estimation : Scope  NumInputPorts=2
  Bus Selector : BusSelector  OutputSignals=Wheel position (rad) [2],Wheel speed (rad/s) [2],Motor Cmd (Volts) [2],Acceleration (m/s/s) [3],Gyroscope (rad/s) [3],Current (Amps) [2],Battle (Volts),Body Speeds Measured (m/s; rad/s) [2]
  Bus Selector1 : BusSelector  OutputSignals=ranges_scan,angles_scan
  Bus Selector3 : BusSelector  OutputSignals=Body Speeds Measured (m/s; rad/s) [2]
  Bus Selector5 : BusSelector  OutputSignals=pose
  Cmd Voltage : Scope  Commented=on
  Current Sense : Scope  Commented=on
  Encoder : Scope  Commented=on
  Gyroscope : Scope  Commented=on
  New Scan : quarc_library/Sinks/Figures/Polar Figure  figure_mode=Use figure window  figure_tag=figure1  axes_tag=axes1  plot_mode=Frame-based  minimum_rho=0  maximum_rho=4  minimum_theta=0  maximum_theta=360  zero_location=top  direction=counterclockwise  buffer_size=2  update_rate=1  sample_time=-1  initial_position="1290   566   484   448"  initial_visibility=off  line1_style=None  line1_width=0.5  line1_color=[0 0 0]  marker1=Point (.)  marker1_size=6  marker1_edge_color=[0 0 0]  marker1_face_color=[0 0 0]  line2_style=Solid line (-)  line2_width=0.5  line2_color=[0.85098 0.32549 0.0980392]  marker2=None  marker2_size=6  marker2_edge_color=[0.85098 0.32549 0.0980392]  marker2_face_color=[0.85098 0.32549 0.0980392]  line3_style=Solid line (-)  line3_width=0.5  line3_color=[0.929412 0.694118 0.12549]  marker3=None  marker3_size=6  marker3_edge_color=[0.929412 0.694118 0.12549]  marker3_face_color=[0.929412 0.694118 0.12549]  line4_style=Solid line (-)  line4_width=0.5  line4_color=[0.494118 0.184314 0.556863]  marker4=None  marker4_size=6  marker4_edge_color=[0.494118 0.184314 0.556863]  marker4_face_color=[0.494118 0.184314 0.556863]  line5_style=Solid line (-)  line5_width=0.5  line5_color=[0.466667 0.67451 0.188235]  marker5=None  marker5_size=6  marker5_edge_color=[0.466667 0.67451 0.188235]  marker5_face_color=[0.466667 0.67451 0.188235]
      settings: SourceProductName=QUARC Targets
  Pose estimate : Scope
  Rate Transition : RateTransition  OutPortSampleTime=lidarStepSize
  Tachometer : Scope  Commented=on
  wires:
  Bus Selector3/1 -> Body Speed estimate pre and post state estimation/2  "<Body Speeds Measured (m/s; rad/s) [2]>"
  Bus Selector/7 -> Battery Sense/1  "<Battle (Volts)>"
  Bus Selector/8 -> Body Speed estimate pre and post state estimation/1  "<Body Speeds Measured (m/s; rad/s) [2]>"
  Bus Selector/6 -> Current Sense/1  "<Current (Amps) [2]>"
  Bus Selector/2 -> Tachometer/1  "<Wheel speed (rad/s) [2]>"
  Bus Selector5/1 -> Pose estimate/1  "<pose>"
  Bus Selector/3 -> Cmd Voltage/1  "<Motor Cmd (Volts) [2]>"
  Bus Selector/1 -> Encoder/1  "<Wheel position (rad) [2]>"
  Bus Selector/5 -> Gyroscope/1  "<Gyroscope (rad/s) [3]>"
  Bus Selector/4 -> Accelerometer/1  "<Acceleration (m/s/s) [3]>"
  Original QBot Data Bus/1 -> Bus Selector/1
  Modified QBot Data Bus/1 -> Bus Selector3/1
  Bus Selector1/2 -> New Scan/2  "<angles_scan>"
  Modified Lidar Data Bus/1 -> Rate Transition/1, Bus Selector5/1
  Bus Selector1/1 -> New Scan/1  "<ranges_scan>"
  Rate Transition/1 -> Bus Selector1/1

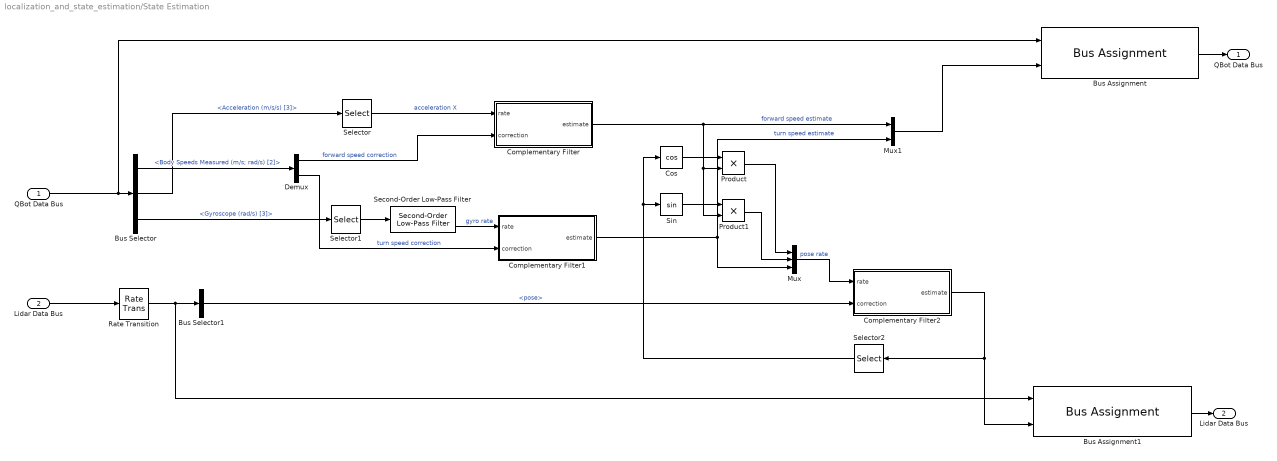
== system localization_and_state_estimation/State Estimation ==
  "QBot Data Bus " : Inport
  "Lidar Data Bus " : Inport  Port=2
  Bus Assignment : BusAssignment  AssignedSignals=Body Speeds Measured (m/s; rad/s) [2]
  Bus Assignment1 : BusAssignment  AssignedSignals=pose
  Bus Selector : BusSelector  OutputSignals=Body Speeds Measured (m/s; rad/s) [2],Acceleration (m/s/s) [3],Gyroscope (rad/s) [3]
  Bus Selector1 : BusSelector  OutputSignals=pose
  Complementary Filter : Subsystem
  Complementary Filter1 : Subsystem
  Complementary Filter2 : Subsystem
  Cos : Trigonometry  Operator=cos
  Demux : Demux  Outputs=2
  Mux : Mux  Inputs=3
  Mux1 : Mux  Inputs=2
  Product : Product
  Product1 : Product
  Rate Transition : RateTransition
  Second-Order Low-Pass Filter : quarc_library/Continuous/Second-Order Low-Pass Filter  params_source=Internal (dialog parameters)  input_width=50  input_zeta=1  input_init=0
  Selector : Selector  InputPortWidth=3  IndexOptions=Index vector (dialog)  Indices=1  OutputSizes=1
  Selector1 : Selector  InputPortWidth=3  IndexOptions=Index vector (dialog)  Indices=3  OutputSizes=1
  Selector2 : Selector  InputPortWidth=3  IndexOptions=Index vector (dialog)  Indices=3  OutputSizes=1
  Sin : Trigonometry
  QBot Data Bus : Outport
  Lidar Data Bus : Outport  Port=2
  wires:
  "QBot Data Bus "/1 -> Bus Assignment/1, Bus Selector/1
  "Lidar Data Bus "/1 -> Rate Transition/1
  Bus Selector/2 -> Selector/1  "<Acceleration (m/s/s) [3]>"
  Selector/1 -> Complementary Filter/1(rate)  "acceleration X"
  Demux/1 -> Complementary Filter/2(correction)  "forward speed correction"
  Complementary Filter/1(estimate) -> Mux1/1, Product1/2, Product/2  "forward speed estimate"
  Bus Selector/3 -> Selector1/1  "<Gyroscope (rad/s) [3]>"
  Selector1/1 -> Second-Order Low-Pass Filter/1
  Second-Order Low-Pass Filter/2 -> Complementary Filter1/1(rate)  "gyro rate"
  Demux/2 -> Complementary Filter1/2(correction)  "turn speed correction"
  Complementary Filter1/1(estimate) -> Mux1/2, Mux/3  "turn speed estimate"
  Bus Selector1/1 -> Complementary Filter2/2(correction)  "<pose>"
  Cos/1 -> Product/1
  Sin/1 -> Product1/1
  Complementary Filter2/1(estimate) -> Bus Assignment1/2, Selector2/1
  Selector2/1 -> Sin/1, Cos/1
  Product1/1 -> Mux/2
  Product/1 -> Mux/1
  Mux/1 -> Complementary Filter2/1(rate)  "pose rate"
  Bus Selector/1 -> Demux/1  "<Body Speeds Measured (m/s; rad/s) [2]>"
  Mux1/1 -> Bus Assignment/2
  Bus Assignment/1 -> QBot Data Bus/1
  Bus Assignment1/1 -> Lidar Data Bus/1
  Rate Transition/1 -> Bus Assignment1/1, Bus Selector1/1

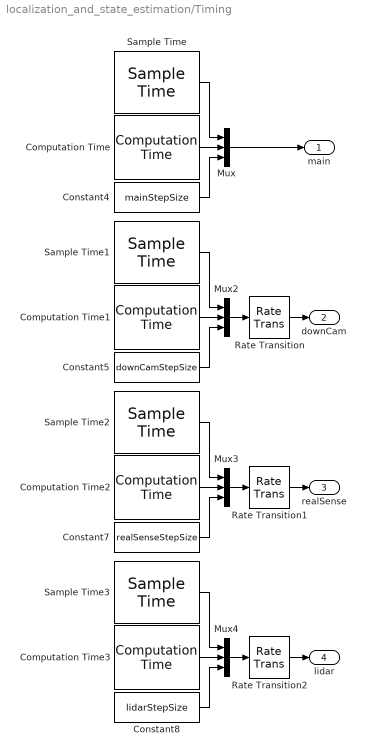
== system localization_and_state_estimation/Timing ==
  Computation Time : quarc_library/Sources/Time/Computation Time  sample_time=mainStepSize  use_model=on  use_cpu_time=off
  Computation Time1 : quarc_library/Sources/Time/Computation Time  sample_time=downCamStepSize  use_model=on  use_cpu_time=off
  Computation Time2 : quarc_library/Sources/Time/Computation Time  sample_time=realSenseStepSize  use_model=on  use_cpu_time=off
  Computation Time3 : quarc_library/Sources/Time/Computation Time  sample_time=lidarStepSize  use_model=on  use_cpu_time=off
  Constant4 : Constant  Value=mainStepSize
  Constant5 : Constant  Value=downCamStepSize
  Constant7 : Constant  Value=realSenseStepSize
  Constant8 : Constant  Value=lidarStepSize
  Mux{,2..4} (4 alike) : Mux  Inputs=3
  Rate Transition : RateTransition
  Rate Transition1 : RateTransition
  Rate Transition2 : RateTransition
  Sample Time : quarc_library/Sources/Time/Sample Time  Priority=-99  sample_time=mainStepSize
  Sample Time1 : quarc_library/Sources/Time/Sample Time  Priority=-99  sample_time=downCamStepSize
  Sample Time2 : quarc_library/Sources/Time/Sample Time  Priority=-99  sample_time=realSenseStepSize
  Sample Time3 : quarc_library/Sources/Time/Sample Time  Priority=-99  sample_time=lidarStepSize
  main : Outport
  downCam : Outport  Port=2
  realSense : Outport  Port=3
  lidar : Outport  Port=4
  wires:
  Rate Transition1/1 -> realSense/1
  Computation Time2/1 -> Mux3/2
  Constant5/1 -> Mux2/3
  Mux4/1 -> Rate Transition2/1
  Computation Time/1 -> Mux/2
  Sample Time/1 -> Mux/1
  Constant8/1 -> Mux4/3
  Sample Time1/1 -> Mux2/1
  Mux3/1 -> Rate Transition1/1
  Computation Time1/1 -> Mux2/2
  Constant4/1 -> Mux/3
  Mux2/1 -> Rate Transition/1
  Computation Time3/1 -> Mux4/2
  Sample Time2/1 -> Mux3/1
  Constant7/1 -> Mux3/3
  Sample Time3/1 -> Mux4/1
  Rate Transition/1 -> downCam/1
  Rate Transition2/1 -> lidar/1
  Mux/1 -> main/1

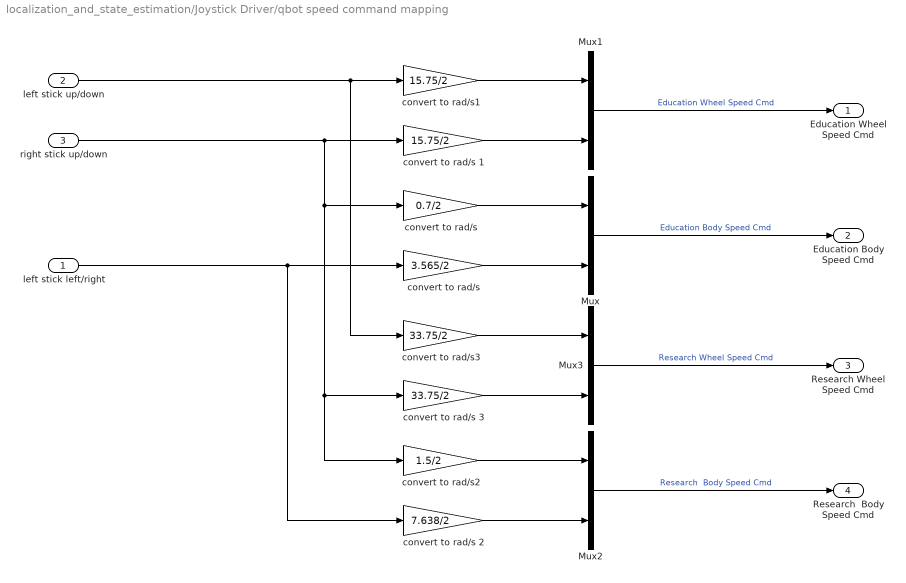
== system localization_and_state_estimation/Joystick Driver/qbot speed command mapping ==
  left stick left/right : Inport
  left stick up/down : Inport  Port=2
  right stick up/down : Inport  Port=3
  Mux{,1..3} (4 alike) : Mux  Inputs=2
  convert to rad/s : Gain  Gain=0.7/2
  "convert to rad/s " : Gain  Gain=3.565/2
  convert to rad/s 1 : Gain  Gain=15.75/2
  convert to rad/s 2 : Gain  Gain=7.638/2
  convert to rad/s 3 : Gain  Gain=33.75/2
  convert to rad/s1 : Gain  Gain=15.75/2
  convert to rad/s2 : Gain  Gain=1.5/2
  convert to rad/s3 : Gain  Gain=33.75/2
  Education Wheel Speed Cmd : Outport
  Education Body Speed Cmd : Outport  Port=2
  Research Wheel Speed Cmd : Outport  Port=3
  Research  Body Speed Cmd : Outport  Port=4
  wires:
  convert to rad/s/1 -> Mux/1
  Mux/1 -> Education Body Speed Cmd/1  "Education Body Speed Cmd"
  left stick left/right/1 -> convert to rad/s 2/1, "convert to rad/s "/1
  convert to rad/s2/1 -> Mux2/1
  left stick up/down/1 -> convert to rad/s3/1, convert to rad/s1/1
  right stick up/down/1 -> convert to rad/s 3/1, convert to rad/s2/1, convert to rad/s/1, convert to rad/s 1/1
  "convert to rad/s "/1 -> Mux/2
  convert to rad/s 3/1 -> Mux3/2
  convert to rad/s3/1 -> Mux3/1
  convert to rad/s 2/1 -> Mux2/2
  convert to rad/s 1/1 -> Mux1/2
  convert to rad/s1/1 -> Mux1/1
  Mux3/1 -> Research Wheel Speed Cmd/1  "Research Wheel Speed Cmd"
  Mux1/1 -> Education Wheel Speed Cmd/1  "Education Wheel Speed Cmd"
  Mux2/1 -> Research  Body Speed Cmd/1  "Research  Body Speed Cmd"

== system localization_and_state_estimation/Lidar & Localization/Freeze scan for reference ==
  ranges_c : Inport
  In2 : Inport  Port=2
  In3 : Inport  Port=3
  Trigger : TriggerPort  VariantControl=(inherit)  InitialTriggerSignalState=zero
  Out1 : Outport
  Out2 : Outport  Port=2
  Out3 : Outport  Port=3
  wires:
  ranges_c/1 -> Out1/1
  In2/1 -> Out2/1
  In3/1 -> Out3/1

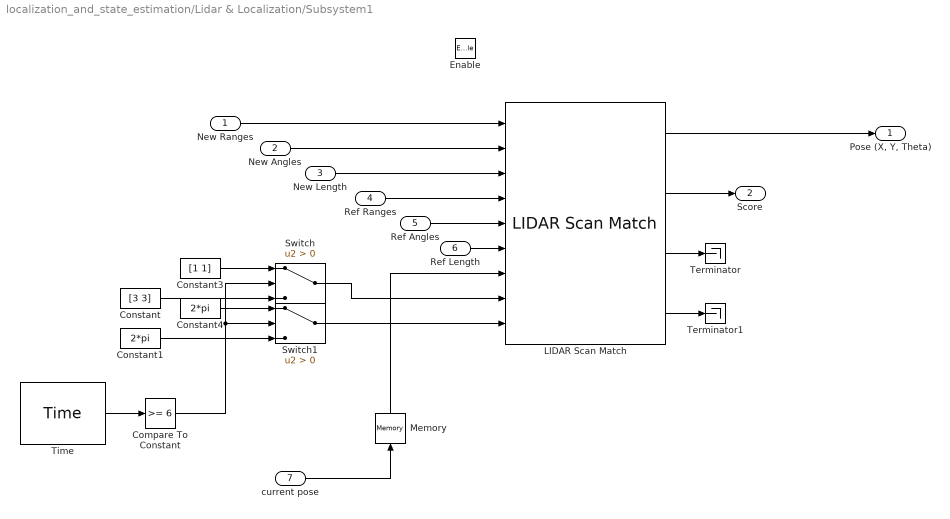
== system localization_and_state_estimation/Lidar & Localization/Subsystem1 ==
  New Ranges : Inport
  New Angles : Inport  Port=2
  New Length : Inport  Port=3
  Ref Ranges : Inport  Port=4
  Ref Angles : Inport  Port=5
  Ref Length : Inport  Port=6
  current pose : Inport  Port=7
  Enable : EnablePort
  Compare To Constant : simulink/Logic and Bit Operations/Compare To Constant  relop=>=  const=6  OutDataTypeStr=boolean
  Constant : Constant  Value=[3 3]
  Constant1 : Constant  Value=2*pi
  Constant3 : Constant  Value=[1 1]
  Constant4 : Constant  Value=2*pi
  LIDAR Scan Match : quarc_library/Image Processing/Generic/LIDAR Scan Match  mode=Fixed input with size  resolution=50  max_range=4  use_initial_pose=on
      settings: SourceProductName=QUARC Targets
  Memory : Memory  InitialCondition=[0 0 0]  InheritSampleTime=on
  Switch : Switch  Criteria=u2 > Threshold  SaturateOnIntegerOverflow=off  InputSameDT=off
  Switch1 : Switch  Criteria=u2 > Threshold  SaturateOnIntegerOverflow=off  InputSameDT=off
  Terminator : Terminator
  Terminator1 : Terminator
  Time : quarc_library/Sources/Time/Time  time_source=Wall clock  sample_time=lidarStepSize
  "Pose (X, Y, Theta)" : Outport
  Score : Outport  Port=2
  wires:
  Ref Ranges/1 -> LIDAR Scan Match/4
  LIDAR Scan Match/2 -> Score/1
  New Angles/1 -> LIDAR Scan Match/2
  Ref Length/1 -> LIDAR Scan Match/6
  LIDAR Scan Match/1 -> "Pose (X, Y, Theta)"/1
  Ref Angles/1 -> LIDAR Scan Match/5
  New Ranges/1 -> LIDAR Scan Match/1
  New Length/1 -> LIDAR Scan Match/3
  LIDAR Scan Match/3 -> Terminator/1
  LIDAR Scan Match/4 -> Terminator1/1
  Memory/1 -> LIDAR Scan Match/7
  Constant/1 -> Switch/3
  Constant1/1 -> Switch1/3
  Time/1 -> Compare To Constant/1
  Compare To Constant/1 -> Switch/2, Switch1/2
  Constant3/1 -> Switch/1
  Constant4/1 -> Switch1/1
  Switch1/1 -> LIDAR Scan Match/9
  Switch/1 -> LIDAR Scan Match/8
  current pose/1 -> Memory/1

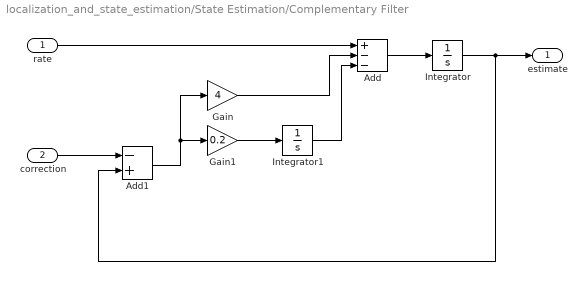
== system localization_and_state_estimation/State Estimation/Complementary Filter ==
  rate : Inport
  correction : Inport  Port=2
  Add : Sum  Inputs=+--
  Add1 : Sum  Inputs=-+
  Gain : Gain  Gain=4
  Gain1 : Gain  Gain=0.2
  Integrator : Integrator
  Integrator1 : Integrator
  estimate : Outport
  wires:
  Integrator/1 -> Add1/2, estimate/1
  Add/1 -> Integrator/1
  rate/1 -> Add/1
  correction/1 -> Add1/1
  Gain1/1 -> Integrator1/1
  Integrator1/1 -> Add/3
  Gain/1 -> Add/2
  Add1/1 -> Gain/1, Gain1/1

== system localization_and_state_estimation/State Estimation/Complementary Filter1 ==
  rate : Inport
  correction : Inport  Port=2
  Add : Sum  Inputs=+--
  Add1 : Sum  Inputs=-+
  Gain : Gain  Gain=4
  Gain1 : Gain  Gain=0.2
  Integrator : Integrator
  Integrator1 : Integrator
  estimate : Outport
  wires:
  Add1/1 -> Gain1/1, Gain/1
  Gain/1 -> Add/2
  Integrator1/1 -> Add/3
  Gain1/1 -> Integrator1/1
  correction/1 -> Add1/1
  rate/1 -> Add/1
  Add/1 -> Integrator/1
  Integrator/1 -> estimate/1, Add1/2

== system localization_and_state_estimation/State Estimation/Complementary Filter2 ==
  rate : Inport
  correction : Inport  Port=2
  Add : Sum  Inputs=+--
  Add1 : Sum  Inputs=-+
  Gain : Gain  Gain=4
  Gain1 : Gain  Gain=0.2
  Integrator : Integrator
  Integrator1 : Integrator
  estimate : Outport
  wires:
  Integrator/1 -> Add1/2, estimate/1
  Add/1 -> Integrator/1
  rate/1 -> Add/1
  correction/1 -> Add1/1
  Gain1/1 -> Integrator1/1
  Integrator1/1 -> Add/3
  Gain/1 -> Add/2
  Add1/1 -> Gain/1, Gain1/1

== matlab function localization_and_state_estimation/Obstacle Detection via Lidar/MATLAB Function ==
  data: ranges input; plottingRanges output; angles input; safetyThreshold input; turnSpd input; plottingAngles output; turnSpeedGain input; minThreshold input; obstacleNumPoints input; obstacleFlag output
function [plottingRanges, plottingAngles, obstacleFlag] = detect_obstacle(ranges, angles, safetyThreshold, turnSpd, turnSpeedGain, minThreshold, obstacleNumPoints)

    halfNumPoints = 205;
    quarterNumPoints = round(halfNumPoints/2);
    
    % Grab the first half of ranges and angles representing 180 degrees
    frontRanges = ranges(1:halfNumPoints);
    frontAngles = angles(1:halfNumPoints);
    
    % Starting index in top half          1     West
    % Mid point in west quadrant         51     North-west
    % Center index in top half          102     North
    % Mid point in east quadrant     51+102     North-east
    % Ending index in top half          205     East
    
    % Normalize turn speed from -1 to 1
    normalizedTurnSpeed = turnSpd/3.564;
    
    % Find starting index to select quarterNumPoints
    startingIndex = round(quarterNumPoints/2) -  round((halfNumPoints/8)*turnSpeedGain*normalizedTurnSpeed);
    if startingIndex < 1
        startingIndex = 1;
    elseif startingIndex > 102
        startingIndex = 102;
    end
    
    % Pick quarterNumPoints in ranges and angles from the front half
    % this will be the region you monitor for obstacles
    monitorRanges = frontRanges(startingIndex:startingIndex+quarterNumPoints);
    monitorAngles = frontAngles(startingIndex:startingIndex+quarterNumPoints);
    
    % At angles corresponding to monitorAngles, pick uniform ranges based on
    % a safety threshold
    safetyAngles = monitorAngles;
    safetyRanges = safetyThreshold*monitorRanges./monitorRanges;

    % Total number of obstacles detected between 
    % minThreshold & safetyThreshold
    totalObstaclePoints = sum((monitorRanges < safetyThreshold).*(monitorRanges > minThreshold));
    if totalObstaclePoints > obstacleNumPoints
        obstacleFlag = 1;
    else
        obstacleFlag = 0;
    end
    
    % Lidar Ranges and Angles for plotting (both scan & safety zone)
    plottingRanges = [monitorRanges; safetyRanges];
    plottingAngles = [monitorAngles; safetyAngles];

end

== matlab function localization_and_state_estimation/Joystick Driver/MATLAB Function ==
  data: u input; N output; S output; E output; W output
function [N, S, E, W] = fcn(u)

N = 0;
S = 0;
E = 0;
W = 0;

switch u
    case 0
        N = 1;
    case 3.142
        S = 1;
    case 4.712
        W = 1;
    case 1.571
        E = 1;
    case 3.927
        S = 1;
        W = 1;
    case 2.356
        S = 1;
        E = 1;
    case 0.7854
        N = 1;
        E = 1;
    case 5.498
        N = 1;
        W = 1;
end

== matlab function localization_and_state_estimation/QBot Hardware/Differential Drive Forward Velocity Kinematics ==
  data: wL input; vC output; wR input; Omega output
function [vC , Omega] = forKin(wL, wR)

% calculate wheel angular velocities
wheelRadius = 3.5*0.0254/2;

vR = wR * wheelRadius;
vL = wL * wheelRadius;

% wheelbase
d=0.3928; 

% calculate wheel linear velocities
vC = (vR + vL)/2;
Omega = (vR - vL)/d;

== matlab function localization_and_state_estimation/Lidar & Localization/Adjust for Center of Measurement ==
  data: lidar_position input; ranges input; ranges_c output; angles input; angles_c output
function [ranges_c,angles_c] = correct_lidar(lidar_position, ranges,angles)

% Convert lidar data from polar into cartesian, and add lidar position
x = ranges.*cos(angles) + lidar_position(1);
y = ranges.*sin(angles) + lidar_position(2);

% Convert back into polar coordinates
ranges_c = sqrt(x.^2 + y.^2);
angles_c = atan2(y, x);

end
